simulink model "untitled"  (R2017b)
settings: Solver=ode45  StartTime=0.0  StopTime=100000  MaxStep=0.01  RelTol=1e-3  EnableMultiTasking=on
values from neighbouring files (symbols this model uses):
  a1 = -0.2074    [equli_fh.m]    (also in reentry_conrridor.m; traj2_sim_init.m)
  a2 = 0.029244    [equli_fh.m]    (also in reentry_conrridor.m; traj2_sim_init.m)
  b1 = 0.06304    [reentry_conrridor.m]    (also in traj2_sim_init.m)
  b2 = 0.6214    [reentry_conrridor.m]    (also in traj2_sim_init.m)
  g0 = 9.81    [equli_fh.m]    (also in reentry_conrridor.m; traj2_sim_init.m)
  hs = 7320    [equli_fh.m]    (also in traj2_sim_init.m)
  mass = 2e4    (= 20000)    [equli_fh.m]    (also in reentry_conrridor.m; traj2_sim_init.m)
  Re = 6378145    [equli_fh.m]    (also in reentry_conrridor.m; traj2_sim_init.m)
  rho0 = 1.225    [equli_fh.m]    (also in reentry_conrridor.m; traj2_sim_init.m)
  sref = 95    [equli_fh.m]    (also in reentry_conrridor.m; traj2_sim_init.m)
settings Model: Creator=ztyab  LastModifiedBy=ztyab
settings DataIOCC: SaveFormat=Array
settings OptimizationCC: LifeSpan=inf
settings DebuggingCC: SolverPrmCheckMsg=warning  SFUnexpectedBacktrackingDiag=warning  SFNoUnconditionalDefaultTransitionDiag=warning  SFExecutionAtInitializationDiag=none
settings HardwareCC: ProdBitPerPointer=32  ProdBitPerSizeT=32  ProdBitPerPtrDiffT=32  ProdLargestAtomicFloat=None  ProdIntDivRoundTo=Undefined  ProdEndianess=Unspecified  ProdWordSize=32  ProdHWDeviceType=32-bit Generic
settings ModelReferenceCC: PropagateSignalLabelsOutOfModel=off
settings CodeAppCC: StateflowObjectComments=on
settings GRTTargetCC: TargetLangStandard=C89/C90 (ANSI)  GeneratePreprocessorConditionals=Disable all
settings ConfigComp: CovMetricSettings=dw  CovHtmlReporting=on  CovSaveCumulativeToWorkspaceVar=on  CovSaveSingleToWorkspaceVar=on  CovExternalEMLEnable=off  CovSFcnEnable=off

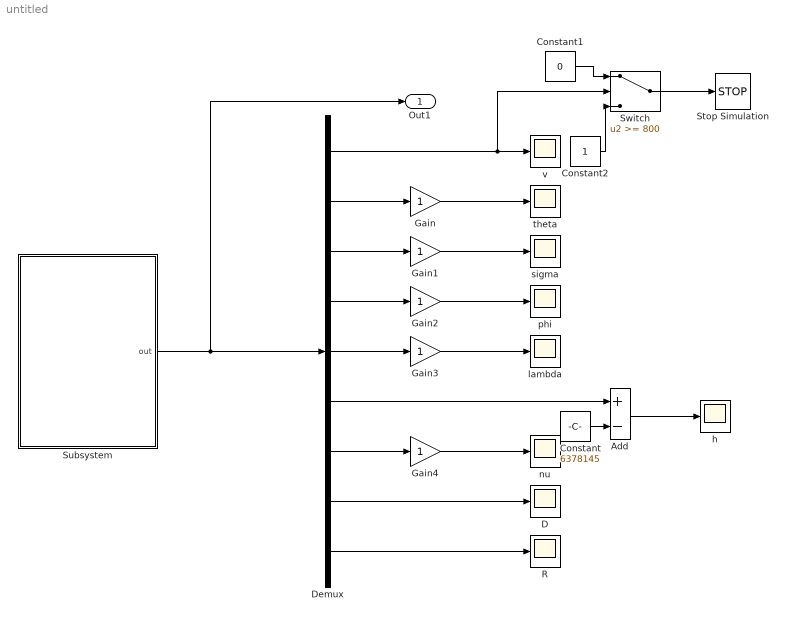
== system untitled ==
  Add : Sum  Inputs=+-
  Constant : Constant  Value=6378145
  Constant1 : Constant  Value=0
  Constant2 : Constant
  D : Scope
  Demux : Demux  Outputs=9
  Gain{,1..4} (5 alike) : Gain
  R : Scope
  Stop Simulation : Stop
  Subsystem : Subsystem
  Switch : Switch  Threshold=800
  h : Scope
  lambda : Scope
  nu : Scope
  phi : Scope
  sigma : Scope
  theta : Scope
  v : Scope
  Out1 : Outport
  wires:
  Subsystem/1(out) -> Out1/1, Demux/1
  Demux/1 -> Switch/2, v/1
  Demux/2 -> Gain/1
  Gain/1 -> theta/1
  Gain1/1 -> sigma/1
  Demux/3 -> Gain1/1
  Gain2/1 -> phi/1
  Demux/4 -> Gain2/1
  Gain3/1 -> lambda/1
  Demux/5 -> Gain3/1
  Demux/6 -> Add/1
  Constant/1 -> Add/2
  Add/1 -> h/1
  Gain4/1 -> nu/1
  Demux/7 -> Gain4/1
  Demux/8 -> D/1
  Demux/9 -> R/1
  Constant1/1 -> Switch/1
  Constant2/1 -> Switch/3
  Switch/1 -> Stop Simulation/1

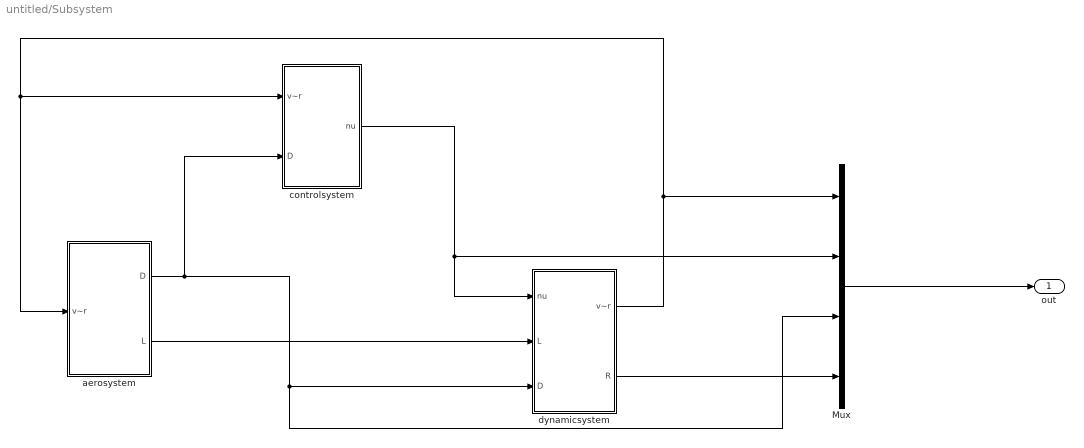
== system untitled/Subsystem ==
  Mux : Mux
  aerosystem : Subsystem
  controlsystem : Subsystem
  dynamicsystem : Subsystem
  out : Outport
  wires:
  dynamicsystem/1(v~r) -> Mux/1, aerosystem/1(v~r), controlsystem/1(v~r)
  controlsystem/1(nu) -> Mux/2, dynamicsystem/1(nu)
  aerosystem/2(L) -> dynamicsystem/2(L)
  aerosystem/1(D) -> dynamicsystem/3(D), Mux/3, controlsystem/2(D)
  Mux/1 -> out/1
  dynamicsystem/2(R) -> Mux/4

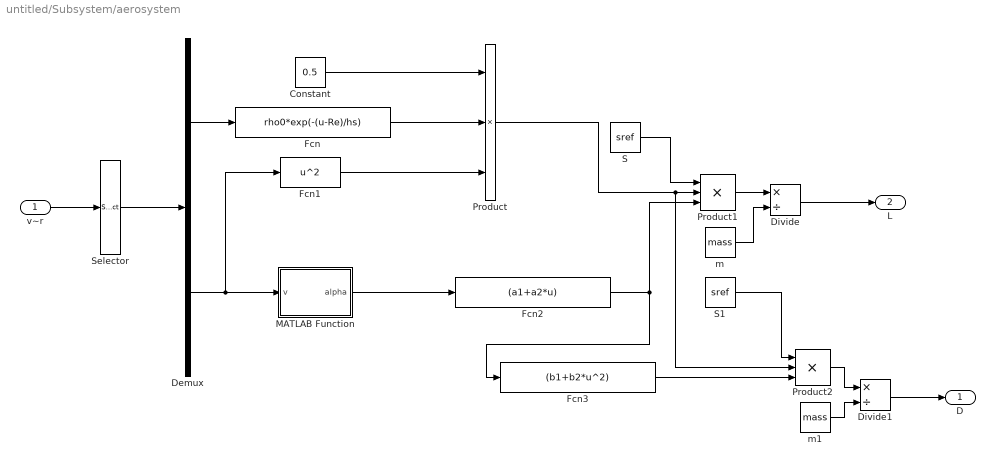
== system untitled/Subsystem/aerosystem ==
  v~r : Inport
  Constant : Constant  Value=0.5
  Demux : Demux  Outputs=2
  Divide : Product  Inputs=*/
  Divide1 : Product  Inputs=*/
  Fcn : Fcn  Expr=rho0*exp(-(u-Re)/hs)
  Fcn1 : Fcn  Expr=u^2
  Fcn2 : Fcn  Expr=(a1+a2*u)
  Fcn3 : Fcn  Expr=(b1+b2*u^2)
  MATLAB Function : MATLAB Function  TreatAsAtomicUnit=on
  Product : Product  Inputs=3
  Product1 : Product  Inputs=3
  Product2 : Product  Inputs=3
  S : Constant  Value=sref
  S1 : Constant  Value=sref
  Selector : Selector  InputPortWidth=6  IndexOptions=Index vector (dialog)  Indices=[6 1]  OutputSizes=1
  m : Constant  Value=mass
  m1 : Constant  Value=mass
  D : Outport
  L : Outport  Port=2
  wires:
  m/1 -> Divide/2
  Fcn3/1 -> Product2/3
  m1/1 -> Divide1/2
  Product2/1 -> Divide1/1
  Divide1/1 -> D/1
  Product/1 -> Product2/2, Product1/2
  S1/1 -> Product2/1
  Product1/1 -> Divide/1
  Divide/1 -> L/1
  Selector/1 -> Demux/1
  v~r/1 -> Selector/1
  Constant/1 -> Product/1
  Fcn/1 -> Product/2
  Fcn1/1 -> Product/3
  Demux/1 -> Fcn/1
  Demux/2 -> MATLAB Function/1(v), Fcn1/1
  MATLAB Function/1(alpha) -> Fcn2/1
  Fcn2/1 -> Fcn3/1, Product1/3
  S/1 -> Product1/1

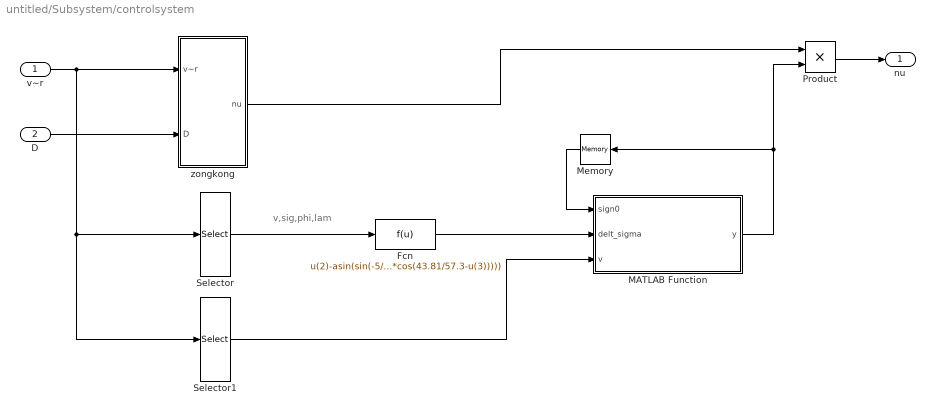
== system untitled/Subsystem/controlsystem ==
  note: v,sig,phi,lam
  v~r : Inport
  D : Inport  Port=2
  Fcn : Fcn  Expr=u(2)-asin(sin(-5/57.3-u(4))/sin(acos(cos(-5/57.3-u(4))*cos(43.81/57.3-u(3)))))
  MATLAB Function : MATLAB Function  TreatAsAtomicUnit=on
  Memory : Memory
  Product : Product
  Selector : Selector  InputPortWidth=6  IndexOptions=Index vector (dialog)  Indices=[1 3 4 5]  OutputSizes=1
  Selector1 : Selector  InputPortWidth=6  IndexOptions=Index vector (dialog)  Indices=[1]  OutputSizes=1
  zongkong : Subsystem
  nu : Outport
  wires:
  Memory/1 -> MATLAB Function/1(sign0)
  Selector/1 -> Fcn/1
  Selector1/1 -> MATLAB Function/3(v)
  Product/1 -> nu/1
  MATLAB Function/1(y) -> Memory/1, Product/2
  Fcn/1 -> MATLAB Function/2(delt_sigma)
  zongkong/1(nu) -> Product/1
  v~r/1 -> Selector1/1, Selector/1, zongkong/1(v~r)
  D/1 -> zongkong/2(D)

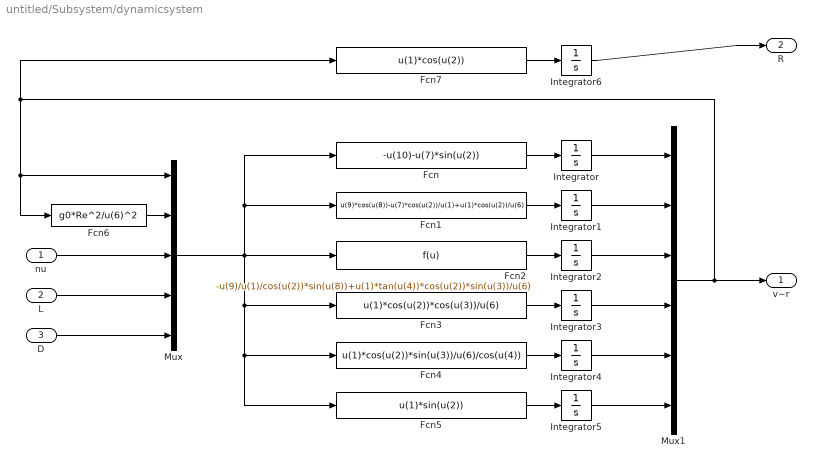
== system untitled/Subsystem/dynamicsystem ==
  nu : Inport
  L : Inport  Port=2
  D : Inport  Port=3
  Fcn : Fcn  Expr=-u(10)-u(7)*sin(u(2))
  Fcn1 : Fcn  Expr=u(9)*cos(u(8))-u(7)*cos(u(2))/u(1)+u(1)*cos(u(2))/u(6)
  Fcn2 : Fcn  Expr=-u(9)/u(1)/cos(u(2))*sin(u(8))+u(1)*tan(u(4))*cos(u(2))*sin(u(3))/u(6)
  Fcn3 : Fcn  Expr=u(1)*cos(u(2))*cos(u(3))/u(6)
  Fcn4 : Fcn  Expr=u(1)*cos(u(2))*sin(u(3))/u(6)/cos(u(4))
  Fcn5 : Fcn  Expr=u(1)*sin(u(2))
  Fcn6 : Fcn  Expr=g0*Re^2/u(6)^2
  Fcn7 : Fcn  Expr=u(1)*cos(u(2))
  Integrator : Integrator  InitialCondition=7800
  Integrator1 : Integrator  InitialCondition=-0.92/57.3
  Integrator2 : Integrator  InitialCondition=51.9/57.3
  Integrator3 : Integrator  InitialCondition=4.79/57.3
  Integrator4 : Integrator  InitialCondition=-85.64/57.3
  Integrator5 : Integrator  InitialCondition=6378145+120000
  Integrator6 : Integrator
  Mux : Mux  Inputs=5
  Mux1 : Mux  Inputs=6
  v~r : Outport
  R : Outport  Port=2
  wires:
  Fcn2/1 -> Integrator2/1
  Integrator2/1 -> Mux1/3
  Integrator3/1 -> Mux1/4
  Integrator4/1 -> Mux1/5
  Integrator6/1 -> R/1
  Fcn/1 -> Integrator/1
  nu/1 -> Mux/3
  D/1 -> Mux/5
  Mux1/1 -> Fcn6/1, Mux/1, Fcn7/1, v~r/1
  Mux/1 -> Fcn/1, Fcn1/1, Fcn5/1, Fcn4/1, Fcn3/1, Fcn2/1
  Integrator/1 -> Mux1/1
  Integrator1/1 -> Mux1/2
  Fcn7/1 -> Integrator6/1
  L/1 -> Mux/4
  Integrator5/1 -> Mux1/6
  Fcn5/1 -> Integrator5/1
  Fcn1/1 -> Integrator1/1
  Fcn3/1 -> Integrator3/1
  Fcn4/1 -> Integrator4/1
  Fcn6/1 -> Mux/2

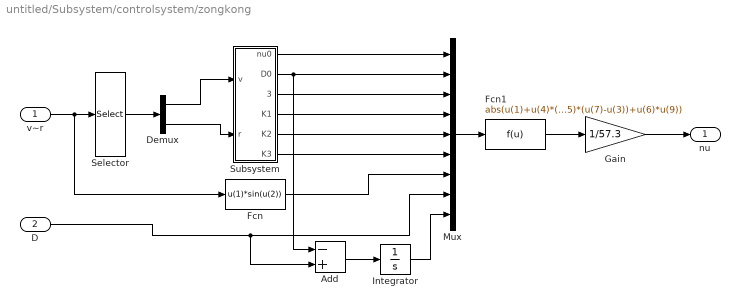
== system untitled/Subsystem/controlsystem/zongkong ==
  v~r : Inport
  D : Inport  Port=2
  Add : Sum  Inputs=-+
  Demux : Demux  Outputs=2
  Fcn : Fcn  Expr=u(1)*sin(u(2))
  Fcn1 : Fcn  Expr=abs(u(1)+u(4)*(u(8)-u(2))+u(5)*(u(7)-u(3))+u(6)*u(9))
  Gain : Gain  Gain=1/57.3
  Integrator : Integrator
  Mux : Mux  Inputs=9
  Selector : Selector  InputPortWidth=6  IndexOptions=Index vector (dialog)  Indices=[1 6]  OutputSizes=1
  Subsystem : Subsystem
  nu : Outport
  wires:
  Fcn1/1 -> Gain/1
  Selector/1 -> Demux/1
  Demux/1 -> Subsystem/1(v)
  Demux/2 -> Subsystem/2(r)
  Gain/1 -> nu/1
  Subsystem/3(diff_h0) -> Mux/3
  Subsystem/5(K2) -> Mux/5
  Integrator/1 -> Mux/9
  Add/1 -> Integrator/1
  Fcn/1 -> Mux/7
  v~r/1 -> Fcn/1, Selector/1
  Subsystem/6(K3) -> Mux/6
  Subsystem/1(nu0) -> Mux/1
  Subsystem/4(K1) -> Mux/4
  D/1 -> Add/2, Mux/8
  Subsystem/2(D0) -> Add/1, Mux/2
  Mux/1 -> Fcn1/1

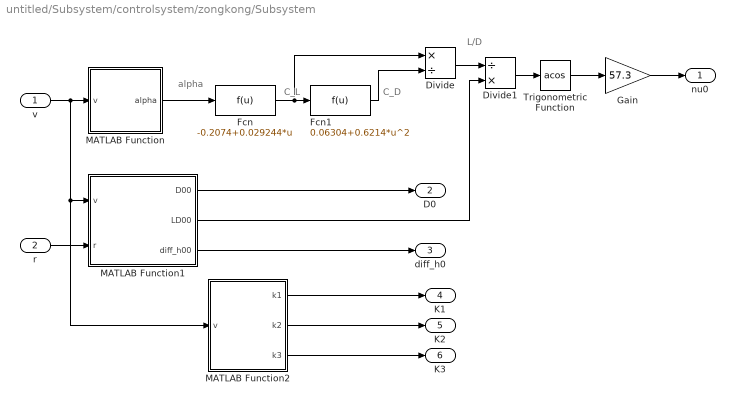
== system untitled/Subsystem/controlsystem/zongkong/Subsystem ==
  note: L/D
  note: C_D
  note: C_L
  note: alpha
  v : Inport
  r : Inport  Port=2
  Divide : Product  Inputs=*/
  Divide1 : Product  Inputs=/*
  Fcn : Fcn  Expr=-0.2074+0.029244*u
  Fcn1 : Fcn  Expr=0.06304+0.6214*u^2
  Gain : Gain  Gain=57.3
  MATLAB Function : MATLAB Function  TreatAsAtomicUnit=on
  MATLAB Function1 : MATLAB Function  TreatAsAtomicUnit=on
  MATLAB Function2 : MATLAB Function  TreatAsAtomicUnit=on
  Trigonometric Function : Trigonometry  Operator=acos
  nu0 : Outport
  D0 : Outport  Port=2
  diff_h0 : Outport  Port=3
  K1 : Outport  Port=4
  K2 : Outport  Port=5
  K3 : Outport  Port=6
  wires:
  Trigonometric Function/1 -> Gain/1
  Fcn1/1 -> Divide/2
  MATLAB Function/1(alpha) -> Fcn/1
  MATLAB Function2/1(k1) -> K1/1
  Gain/1 -> nu0/1
  MATLAB Function1/2(LD00) -> Divide1/2
  MATLAB Function1/1(D00) -> D0/1
  r/1 -> MATLAB Function1/2(r)
  MATLAB Function1/3(diff_h00) -> diff_h0/1
  Divide/1 -> Divide1/1
  v/1 -> MATLAB Function1/1(v), MATLAB Function2/1(v), MATLAB Function/1(v)
  MATLAB Function2/3(k3) -> K3/1
  MATLAB Function2/2(k2) -> K2/1
  Divide1/1 -> Trigonometric Function/1
  Fcn/1 -> Divide/1, Fcn1/1

== matlab function untitled/Subsystem/controlsystem/zongkong/Subsystem/MATLAB Function1 ==
  data: v input; D00 output; r input; LD00 output; diff_h00 output
function [D00,LD00,diff_h00] = stdfcn(v,r)
%#codegen
hs=7320;
g0=9.81;
Re=6378145;
mu=g0*Re^2;
g=mu/r^2;
D=0;
LD0=0;
diff_h0=0;
if v>=750&&v<3300
    D=4.3626+0.0017083*v;
    diff_h0=-hs/v*(2*4.3626+0.0017083*v);
    LD0=g/D*(1-v^2/g/r)-4*hs*4.3626/v^2-hs*0.0017083/v;
elseif v>=3300&&v<5000
    D=10;
    diff_h0=-hs/v*(2*10);
    LD0=g/D*(1-v^2/g/r)-4*hs*D/v^2;
elseif v>=5000&&v<6300
    D=25.38-0.003077*v;
    diff_h0=-hs/v*(2*25.38-0.003077*v);
    LD0=g/D*(1-v^2/g/r)-4*hs*25.38/v^2+hs*0.003077/v;
elseif v>=6300&&v<7400
    D=-7.584+0.006915*v-7.554*10^(-7)*v^2;
    diff_h0=-hs/v*(2*(-7.584)+0.006915*v);
    LD0=g/D*(1-v^2/g/r)-4*hs*(-7.584)/v^2-hs*0.006915/v;  
elseif v>=7400&&v<=7800
    D=185.001-0.04311*v+2.4875*10^(-6)*v^2;
    diff_h0=-hs/v*(2*185.001-0.04311*v);
    LD0=g/D*(1-v^2/g/r)-4*hs*185.001/v^2+hs*0.04311/v; 
end
D00=D;
LD00=LD0;
diff_h00=diff_h0;
end

== matlab function untitled/Subsystem/controlsystem/zongkong/Subsystem/MATLAB Function ==
  data: v input; alpha output
function alpha = fcn1(v)
%#codegen
if v<775
    alpha0=18;
elseif 775<=v&v<4000
    alpha0=18+(v-775)/146;
else
    alpha0=40;
end
alpha=alpha0;
end

== matlab function untitled/Subsystem/controlsystem/MATLAB Function ==
  data: sign0 input; y output; delt_sigma input; v input
function y = fcn(sign0,delt_sigma,v)
%#codegen
delt_sigma1=12/180*pi;
delt_sigma2=20/180*pi;
if (v>=6000)
    if (delt_sigma>delt_sigma1)
        sign=1;
    elseif (delt_sigma<=delt_sigma1)&&(delt_sigma>=-delt_sigma1)
        sign=sign0;
    else 
        sign=-1;
    end
else
    if (delt_sigma>delt_sigma2)
        sign=1;
    elseif (delt_sigma<=delt_sigma2)&&(delt_sigma>=-delt_sigma2)
        sign=sign0;
    else 
        sign=-1;
    end
end
y =sign;
end

== matlab function untitled/Subsystem/aerosystem/MATLAB Function ==
  data: v input; alpha output
function alpha =Alpha_fun(v)
if v<775
    alpha0=18;
elseif 775<=v&v<4000
    alpha0=18+(v-775)/146;
else
    alpha0=40;
end
alpha=alpha0;
end

== matlab function untitled/Subsystem/controlsystem/zongkong/Subsystem/MATLAB Function2 ==
  data: v input; k1 output; k2 output; k3 output
function [k1,k2,k3] = fcn1(v)
%#codegen
if v>=7500
    a1=-70;
    a2=0.6;
    a3=-0.3;
elseif v>=7000&v<7500
    a1=-70;
    a2=1;
    a3=-0.2;
elseif v>=6300&v<7000
    a1=-70;
    a2=1;
    a3=-0.5;
elseif v>=5000&v<6300
    a1=-40;
    a2=0.8;
    a3=-0.8;
elseif v>=4000&v<5000
    a1=-100;
    a2=0.8;
    a3=-0.6;
elseif v>=3500&v<4000
    a1=-150;
    a2=0.2;
    a3=-0.4;
elseif v>=2000&v<3500
    a1=-60;
    a2=0.5;
    a3=-1.2;
else
    a1=-60;
     a2=0.1;
     a2=0.5;
     a3=-2;
     a3=-1.2;
end
k1=a1;
k2=a2;
k3=a3;
end
